simulink model "User_Interface_Unit"  (R2019a)
settings: Solver=ode2  StartTime=0.0  StopTime=inf  FixedStep=0.002  RelTol=1e-3  EnableMultiTasking=on
undefined symbols (not defined in the file): Host
libraries: quarc_library x15, simulink x6
settings Model: Creator=User  LastModifiedBy=mbohra
settings SolverCC: PositivePriorityOrder=on
settings DataIOCC: ReturnWorkspaceOutputs=off
settings DebuggingCC: PregeneratedLibrarySubsystemCodeDiagnostic=none  ArithmeticOperatorsInVariantConditions=warning
settings SFSimCC: SimUseLocalCustomCode=off
settings RTWCC: SystemTargetFile=quarc_linux_nvidia.tlc  TemplateMakefile=quarc_linux_nvidia_tmf  Description=QUARC Linux Nvidia Target  RTWUseLocalCustomCode=off
settings STFCustomTargetCC: TargetLibSuffix=.a  TargetPreCompLibLocation=C:\PROGRA~3\QUARC\lib\2019a\LINUX_~1\release  TargetLangStandard=C99 (ISO)  ConcurrentExecutionCompliant=on  SystemTargetFile=quarc_linux_nvidia.tlc
settings GRTTargetCC: TargetLibSuffix=.a  TargetPreCompLibLocation=C:\PROGRA~3\QUARC\lib\2019a\LINUX_~1\release  ParMdlRefBuildCompliant=off  CompOptLevelCompliant=off  CombineOutputUpdateFcns=off  MatFileLogging=off  CPPClassGenCompliant=off  GRTInterface=on  UseToolchainInfoCompliant=off  ExtMode=on  ExtModeMexFile=quarc_comm  ExtModeMexArgs='-w -d /tmp -uri %u'

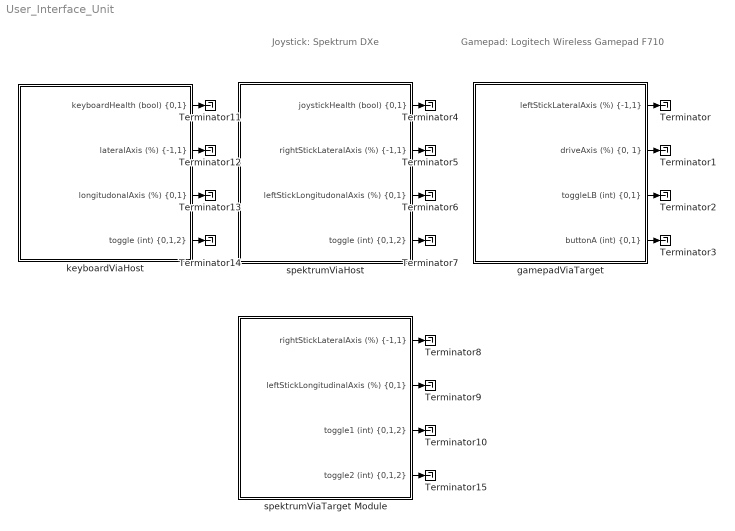
== system User_Interface_Unit ==
  note: Gamepad: Logitech Wireless Gamepad F710
  note: Joystick: Spektrum DXe
  Terminator{,1..15} (16 alike) : Terminator
  gamepadViaTarget : Subsystem
  keyboardViaHost : Subsystem
  spektrumViaHost : Subsystem
  spektrumViaTarget Module : Subsystem
  wires:
  keyboardViaHost/3("longitudonalAxis (%) {0,1}") -> Terminator13/1
  spektrumViaTarget Module/3("toggle1 (int) {0,1,2}") -> Terminator10/1
  spektrumViaHost/2("rightStickLateralAxis (%) {-1,1}") -> Terminator5/1
  spektrumViaTarget Module/2("leftStickLongitudinalAxis (%) {0,1}") -> Terminator9/1
  spektrumViaTarget Module/4("toggle2 (int) {0,1,2}") -> Terminator15/1
  spektrumViaHost/1("joystickHealth (bool) {0,1}") -> Terminator4/1
  spektrumViaTarget Module/1("rightStickLateralAxis (%) {-1,1}") -> Terminator8/1
  spektrumViaHost/3("leftStickLongitudonalAxis (%) {0,1}") -> Terminator6/1
  spektrumViaHost/4("toggle (int) {0,1,2}") -> Terminator7/1
  keyboardViaHost/2("lateralAxis (%) {-1,1}") -> Terminator12/1
  keyboardViaHost/4("toggle (int) {0,1,2}") -> Terminator14/1
  keyboardViaHost/1("keyboardHealth (bool) {0,1}") -> Terminator11/1
  gamepadViaTarget/1("leftStickLateralAxis (%) {-1,1}") -> Terminator/1
  gamepadViaTarget/2("driveAxis (%) {0, 1}") -> Terminator1/1
  gamepadViaTarget/3("toggleLB (int) {0,1}") -> Terminator2/1
  gamepadViaTarget/4("buttonA (int) {0,1}") -> Terminator3/1

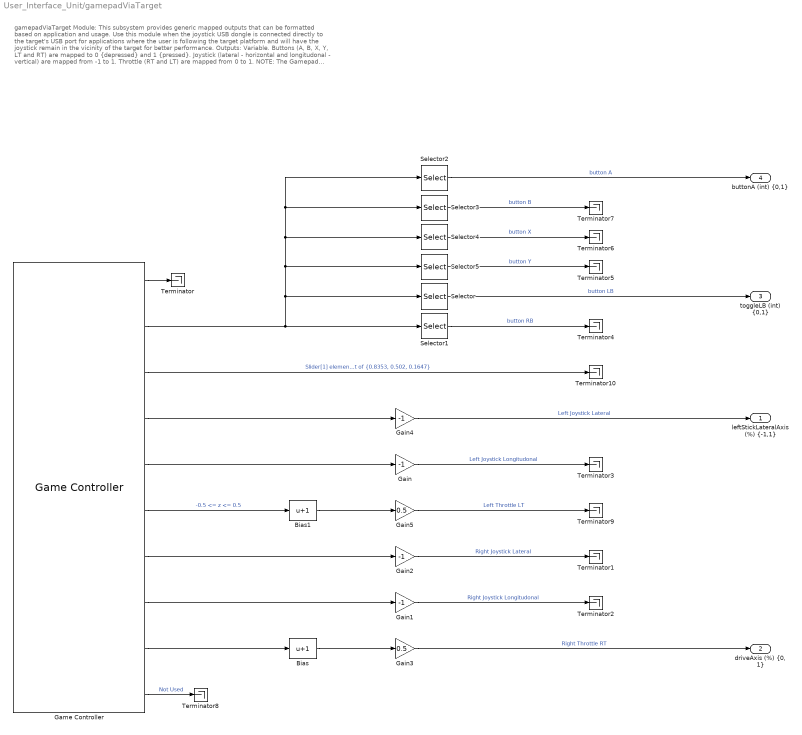
== system User_Interface_Unit/gamepadViaTarget ==
  note: gamepadViaTarget Module:
      |
      | This subsystem provides generic mapped outputs that can be formatted based on application and usage. Use this module when the joystick USB dongle is connected directly to the target's USB port for applications where the user is following the target platform and will have the joystick remain in the vicinity of the target for better performance.
      |
      | Outputs:
      | Variable.
      | Buttons (A, B, X, Y, LT and RT) are mapped to 0 {depressed} and 1 {pressed}.
      | Joystick (lateral - horizontal and longitudonal - vertical) are mapped from -1 to 1.
      | Throttle (RT and LT) are mapped from 0 to 1.
      |
      | NOTE: The Gamepad F710 dongle MUST be plugged into the target's USB port to use this module. Connect the target to a Monitor/Keyboard/Mouse or SSH into the client and run the following command in the terminal:
      | ls -l /dev/input/by-id
      | Find the output with the term ' usb-Logitech_Wireless_Gamepad_F710_XXXXXXX 4-event-joystick ' in it. Find the event number at the end, for example ../event6 , and add 1 to it, for example, 6+1 = 7. Use that as the Controller # in the Game Controller block below.
  Bias : Bias  Bias=1
  Bias1 : Bias  Bias=1
  Gain{,1..2,4} (4 alike) : Gain  Gain=-1
  Gain3 : Gain  Gain=0.5
  Gain5 : Gain  Gain=0.5
  Game Controller : quarc_library/Devices/Peripherals/Target/Game Controller  controller=7  buffer_size=12  deadzone=[]  saturation=[]  sample_time=qc_get_step_size  auto_center=off  enabled=on
      settings: SourceProductName=QUARC Targets
  Selector : Selector  InputPortWidth=32  IndexOptions=Index vector (dialog)  Indices=[5]  OutputSizes=1
  Selector1 : Selector  InputPortWidth=32  IndexOptions=Index vector (dialog)  Indices=[6]  OutputSizes=1
  Selector2 : Selector  InputPortWidth=32  IndexOptions=Index vector (dialog)  Indices=[1]  OutputSizes=1
  Selector3 : Selector  InputPortWidth=32  IndexOptions=Index vector (dialog)  Indices=[2]  OutputSizes=1
  Selector4 : Selector  InputPortWidth=32  IndexOptions=Index vector (dialog)  Indices=[3]  OutputSizes=1
  Selector5 : Selector  InputPortWidth=32  IndexOptions=Index vector (dialog)  Indices=[4]  OutputSizes=1
  Terminator{,1..10} (11 alike) : Terminator
  "leftStickLateralAxis (%) {-1,1}" : Outport
  "driveAxis (%) {0, 1}" : Outport  Port=2
  "toggleLB (int) {0,1}" : Outport  Port=3
  "buttonA (int) {0,1}" : Outport  Port=4
  wires:
  Selector1/1 -> Terminator4/1  "button RB"
  Gain/1 -> Terminator3/1  "Left Joystick Longitudonal"
  Gain1/1 -> Terminator2/1  "Right Joystick Longitudonal"
  Gain2/1 -> Terminator1/1  "Right Joystick Lateral"
  Selector2/1 -> "buttonA (int) {0,1}"/1  "button A"
  Gain4/1 -> "leftStickLateralAxis (%) {-1,1}"/1  "Left Joystick Lateral"
  Gain3/1 -> "driveAxis (%) {0, 1}"/1  "Right Throttle RT"
  Bias/1 -> Gain3/1
  Game Controller/9 -> Bias/1
  Selector/1 -> "toggleLB (int) {0,1}"/1  "button LB"
  Game Controller/2 -> Selector4/1, Selector3/1, Selector2/1, Selector5/1, Selector/1, Selector1/1
  Game Controller/7 -> Gain2/1
  Game Controller/8 -> Gain1/1
  Game Controller/4 -> Gain4/1
  Game Controller/5 -> Gain/1
  Game Controller/1 -> Terminator/1
  Selector3/1 -> Terminator7/1  "button B"
  Selector4/1 -> Terminator6/1  "button X"
  Selector5/1 -> Terminator5/1  "button Y"
  Game Controller/10 -> Terminator8/1  "Not Used"
  Game Controller/6 -> Bias1/1  "-0.5 <= z <= 0.5"
  Bias1/1 -> Gain5/1
  Gain5/1 -> Terminator9/1  "Left Throttle LT"
  Game Controller/3 -> Terminator10/1  "Slider[1] element of {0.8353, 0.502, 0.1647}"

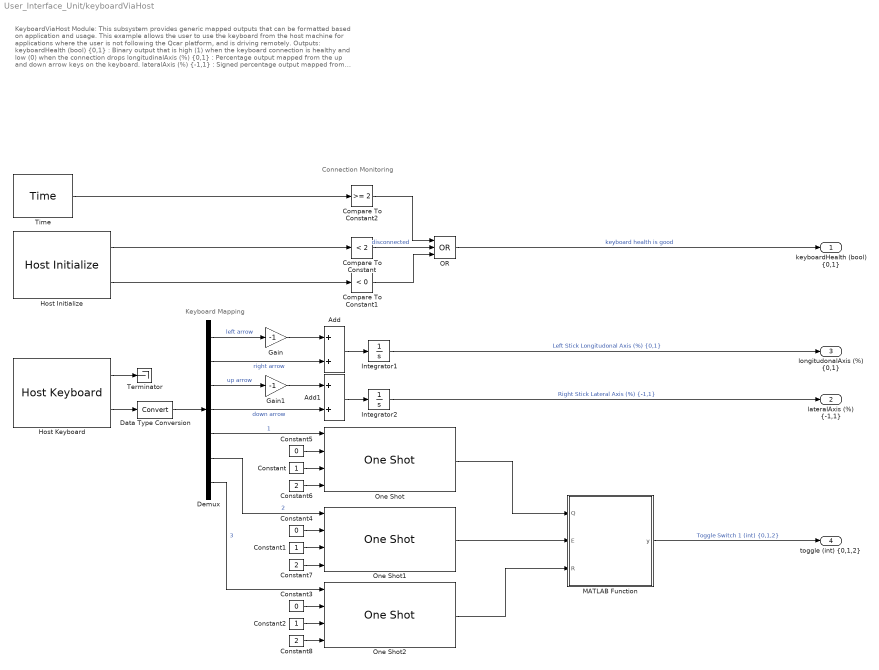
== system User_Interface_Unit/keyboardViaHost ==
  note: Connection Monitoring
  note: KeyboardViaHost Module:
      |
      | This subsystem provides generic mapped outputs that can be formatted based on application and usage. This example allows the user to use the keyboard from the host machine for applications where the user is not following the Qcar platform, and is driving remotely.
      |
      | Outputs:
      | keyboardHealth (bool) {0,1} : Binary output that is high (1) when the keyboard connection is healthy and low (0) when the connection drops
      | longitudinalAxis (%) {0,1} : Percentage output mapped from the up and down arrow keys on the keyboard.
      | lateralAxis (%) {-1,1} : Signed percentage output mapped from the left and right arrow keys on the keyboard.
      | toggle (int) {0,1,2} : 3-state output mapped from the 1, 2, 3 alpha-numeric keys (NOT on the NUMPAD).
      |
      | Note: Holding the arrow keys longer will increase/decrease the value further. Releasing the key will maintain values.
  note: Keyboard Mapping
  Add : Sum
  Add1 : Sum
  Compare To Constant : simulink/Logic and Bit Operations/Compare To Constant  relop=<  const=2  OutDataTypeStr=boolean
  Compare To Constant1 : simulink/Logic and Bit Operations/Compare To Constant  relop=<  const=0  OutDataTypeStr=boolean
  Compare To Constant2 : simulink/Logic and Bit Operations/Compare To Constant  relop=>=  const=2  OutDataTypeStr=boolean
  Constant : Constant
  Constant1 : Constant
  Constant2 : Constant
  Constant3 : Constant  Value=0
  Constant4 : Constant  Value=0
  Constant5 : Constant  Value=0
  Constant6 : Constant  Value=2
  Constant7 : Constant  Value=2
  Constant8 : Constant  Value=2
  Data Type Conversion : DataTypeConversion
  Demux : Demux  Outputs=7
  Gain : Gain  Gain=-1
  Gain1 : Gain  Gain=-1
  Host Initialize : quarc_library/Devices/Peripherals/Host/Host Initialize  object_name=Host-2  uri_source=Use external mode communications  uri=tcpip://localhost:18001  apply_uri_to_all_configs=on  send_buffer_size=1000  receive_buffer_size=1000  thread_priority=0  run_client=on  use_window=off  window_position=[]  sample_time=qc_get_step_size  active=on
      settings: SourceProductName=QUARC Targets
  Host Keyboard : quarc_library/Devices/Peripherals/Host/Host Keyboard  object_name=Host-2  virtual_key="[37  39  40  38  49  50  51]"  sample_time=qc_get_step_size  enabled=on  debug_mode=off
      settings: SourceProductName=QUARC Targets
  Integrator1 : Integrator  LimitOutput=on  UpperSaturationLimit=1  LowerSaturationLimit=0
  Integrator2 : Integrator  LimitOutput=on  UpperSaturationLimit=1  LowerSaturationLimit=-1
  MATLAB Function : MATLAB Function  TreatAsAtomicUnit=on
  OR : Logic  Operator=OR  Inputs=3  IconShape=distinctive  AllPortsSameDT=off  OutDataTypeStr=boolean
  One Shot : quarc_library/Discontinuities/One Shot  trigger_type=Rising edge  redun_pulse=Ignore extraneous pulse  width_source=External input port  pulse_width=100
      settings: SourceProductName=QUARC Targets
  One Shot1 : quarc_library/Discontinuities/One Shot  trigger_type=Rising edge  redun_pulse=Ignore extraneous pulse  width_source=External input port  pulse_width=100
      settings: SourceProductName=QUARC Targets
  One Shot2 : quarc_library/Discontinuities/One Shot  trigger_type=Rising edge  redun_pulse=Ignore extraneous pulse  width_source=External input port  pulse_width=100
      settings: SourceProductName=QUARC Targets
  Terminator : Terminator
  Time : quarc_library/Sources/Time/Time  time_source=Wall clock  sample_time=qc_get_step_size
  "keyboardHealth (bool) {0,1}" : Outport
  "lateralAxis (%) {-1,1}" : Outport  Port=2
  "longitudonalAxis (%) {0,1}" : Outport  Port=3
  "toggle (int) {0,1,2}" : Outport  Port=4
  wires:
  Integrator1/1 -> "longitudonalAxis (%) {0,1}"/1  "Left Stick Longitudonal Axis (%) {0,1}"
  One Shot/1 -> MATLAB Function/1(Q)
  Constant2/1 -> One Shot2/3
  Host Initialize/1 -> Compare To Constant/1
  Constant/1 -> One Shot/3
  Constant6/1 -> One Shot/4
  Demux/2 -> Add/2  "right arrow"
  One Shot1/1 -> MATLAB Function/2(E)
  Compare To Constant/1 -> OR/2  "disconnected"
  One Shot2/1 -> MATLAB Function/3(R)
  Integrator2/1 -> "lateralAxis (%) {-1,1}"/1  "Right Stick Lateral Axis (%) {-1,1}"
  Demux/1 -> Gain/1  "left arrow"
  Constant3/1 -> One Shot2/2
  Constant8/1 -> One Shot2/4
  Host Keyboard/2 -> Data Type Conversion/1
  Gain1/1 -> Add1/1
  OR/1 -> "keyboardHealth (bool) {0,1}"/1  "keyboard health is good"
  Demux/7 -> One Shot2/1  "3"
  Constant4/1 -> One Shot1/2
  Constant1/1 -> One Shot1/3
  Demux/5 -> One Shot/1  "1"
  Compare To Constant2/1 -> OR/1
  Time/1 -> Compare To Constant2/1
  Host Keyboard/1 -> Terminator/1
  Add1/1 -> Integrator2/1
  Gain/1 -> Add/1
  Constant5/1 -> One Shot/2
  Add/1 -> Integrator1/1
  Constant7/1 -> One Shot1/4
  Compare To Constant1/1 -> OR/3
  Data Type Conversion/1 -> Demux/1
  Host Initialize/2 -> Compare To Constant1/1
  MATLAB Function/1(y) -> "toggle (int) {0,1,2}"/1  "Toggle Switch 1 (int) {0,1,2}"
  Demux/3 -> Gain1/1  "up arrow"
  Demux/4 -> Add1/2  "down arrow"
  Demux/6 -> One Shot1/1  "2"

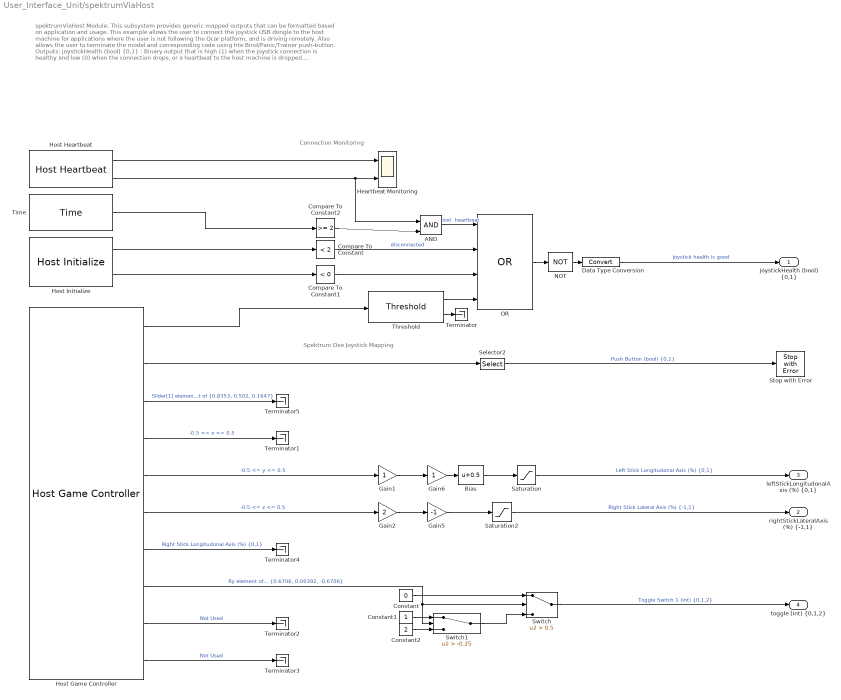
== system User_Interface_Unit/spektrumViaHost ==
  note: Connection Monitoring
  note: Spektrum Dxe Joystick Mapping
  note: spektrumViaHost Module:
      |
      | This subsystem provides generic mapped outputs that can be formatted based on application and usage. This example allows the user to connect the joystick USB dongle to the host machine for applications where the user is not following the Qcar platform, and is driving remotely. Also allows the user to terminate the model and corresponding code using hte Bind/Panic/Trainer push-button.
      |
      | Outputs:
      | joystickHealth (bool) {0,1} : Binary output that is high (1) when the joystick connection is healthy and low (0) when the connection drops, or a heartbeat to the host machine is dropped.
      | leftStickLongitudinalAxis (%) {0,1} : Percentage output mapped from the left stick of the joystick in the longitudinal axis
      | rightStickLateralAxis (%) {-1,1} : Signed percentage output mapped from the right stick of the joystick in the lateral axis
      | toggle (int) {0,1,2} : 3-state output mapped from the joystick's first toggle (labelled Flight Mode)
      |
      | NOTE: The Spektrum Joystick USB Dongle MUST be plugged into the Host PC's USB port to use this module. Open the Host Game Controller block below, and in the Controller number menu, select the one with the SPEKTRUM RECEIVER label next to it.
  AND : Logic  IconShape=distinctive  AllPortsSameDT=off  OutDataTypeStr=boolean
  Bias : Bias  Bias=0.5
  Compare To Constant : simulink/Logic and Bit Operations/Compare To Constant  relop=<  const=2  OutDataTypeStr=boolean
  Compare To Constant1 : simulink/Logic and Bit Operations/Compare To Constant  relop=<  const=0  OutDataTypeStr=boolean
  Compare To Constant2 : simulink/Logic and Bit Operations/Compare To Constant  relop=>=  const=2  OutDataTypeStr=boolean
  Constant : Constant  Value=0
  Constant1 : Constant
  Constant2 : Constant  Value=2
  Data Type Conversion : DataTypeConversion
  Gain1 : Gain
  Gain2 : Gain  Gain=2
  Gain5 : Gain  Gain=-1
  Gain6 : Gain
  Heartbeat Monitoring : Scope  NumInputPorts=2
  Host Game Controller : quarc_library/Devices/Peripherals/Host/Host Game Controller  object_name=Host-1  controller=1  buffer_size=12  deadzone=[]  saturation=[]  sample_time=qc_get_step_size  auto_center=off  enabled=off  debug_mode=off
      settings: SourceProductName=QUARC Targets
  Host Heartbeat : quarc_library/Devices/Peripherals/Host/Host Heartbeat  object_name=Host-1  period=0.1  loss_interval=0.5  sample_time=qc_get_step_size  enabled=off
      settings: SourceProductName=QUARC Targets
  Host Initialize : quarc_library/Devices/Peripherals/Host/Host Initialize  object_name=Host-1  uri_source=Specify via dialog (do not evaluate)  uri=tcpip://%h:18001  apply_uri_to_all_configs=on  send_buffer_size=1000  receive_buffer_size=1000  thread_priority=0  run_client=on  use_window=off  window_position=[]  sample_time=qc_get_step_size  active=on
      settings: AttributesFormatString="\"tcpip://linuxdev:18001\""  SourceProductName=QUARC Targets
  NOT : Logic  Operator=NOT  IconShape=distinctive  AllPortsSameDT=off  OutDataTypeStr=boolean
  OR : Logic  Operator=OR  Inputs=4  IconShape=distinctive  AllPortsSameDT=off  OutDataTypeStr=boolean
  Saturation : Saturate  UpperLimit=1  LowerLimit=0
  Saturation2 : Saturate  UpperLimit=1  LowerLimit=-1
  Selector2 : Selector  InputPortWidth=32  IndexOptions=Index vector (dialog)  Indices=[1]  OutputSizes=1
  Stop with Error : quarc_library/Sinks/Error Handling/Stop with Error  message_type=Fixed error message  message=Emergency Stop Issued
      settings: AttributesFormatString="\"%<message>\""  SourceProductName=QUARC Targets
  Switch : Switch  Criteria=u2 > Threshold  Threshold=0.5
  Switch1 : Switch  Criteria=u2 > Threshold  Threshold=-0.25
  Terminator{,1..5} (6 alike) : Terminator
  Threshold : quarc_library/Discontinuities/Threshold  operator=<=  param_src=Specify via dialog  threshold=0  duration=2
      settings: SourceProductName=QUARC Targets
  Time : quarc_library/Sources/Time/Time  time_source=Wall clock  sample_time=qc_get_step_size
  "joystickHealth (bool) {0,1}" : Outport
  "rightStickLateralAxis (%) {-1,1}" : Outport  Port=2
  "leftStickLongitudonalAxis (%) {0,1}" : Outport  Port=3
  "toggle (int) {0,1,2}" : Outport  Port=4
  wires:
  Constant/1 -> Switch/1
  Host Game Controller/9 -> Terminator2/1  "Not Used"
  Host Game Controller/2 -> Selector2/1
  Host Game Controller/8 -> Switch1/2, Switch/2  "Ry element of {0.6706, 0.00392, -0.6706}"
  Constant1/1 -> Switch1/1
  Switch1/1 -> Switch/3
  Host Game Controller/5 -> Gain1/1  "-0.5 <= y <= 0.5"
  Saturation/1 -> "leftStickLongitudonalAxis (%) {0,1}"/1  "Left Stick Longitudonal Axis (%) {0,1}"
  Compare To Constant2/1 -> AND/2
  Switch/1 -> "toggle (int) {0,1,2}"/1  "Toggle Switch 1 (int) {0,1,2}"
  Bias/1 -> Saturation/1
  Gain5/1 -> Saturation2/1
  Host Heartbeat/2 -> AND/1, Heartbeat Monitoring/2
  Gain1/1 -> Gain6/1
  Saturation2/1 -> "rightStickLateralAxis (%) {-1,1}"/1  "Right Stick Lateral Axis (%) {-1,1}"
  Time/1 -> Compare To Constant2/1
  Host Game Controller/4 -> Terminator1/1  "-0.5 <= x <= 0.5"
  Compare To Constant/1 -> OR/2  "disconnected"
  Host Game Controller/3 -> Terminator5/1  "Slider[1] element of {0.8353, 0.502, 0.1647}"
  Host Game Controller/6 -> Gain2/1  "-0.5 <= z <= 0.5"
  Gain2/1 -> Gain5/1
  Data Type Conversion/1 -> "joystickHealth (bool) {0,1}"/1  "joystick health is good"
  OR/1 -> NOT/1
  Gain6/1 -> Bias/1
  Threshold/1 -> OR/4
  Host Heartbeat/1 -> Heartbeat Monitoring/1
  Host Game Controller/7 -> Terminator4/1  "Right Stick Longitudonal Axis (%) {0,1}"
  AND/1 -> OR/1  "lost  heartbeat"
  Threshold/2 -> Terminator/1
  Host Game Controller/1 -> Threshold/1
  Compare To Constant1/1 -> OR/3
  Host Game Controller/10 -> Terminator3/1  "Not Used"
  Constant2/1 -> Switch1/3
  Host Initialize/2 -> Compare To Constant1/1
  Host Initialize/1 -> Compare To Constant/1
  Selector2/1 -> Stop with Error/1  "Push Button (bool) {0,1}"
  NOT/1 -> Data Type Conversion/1

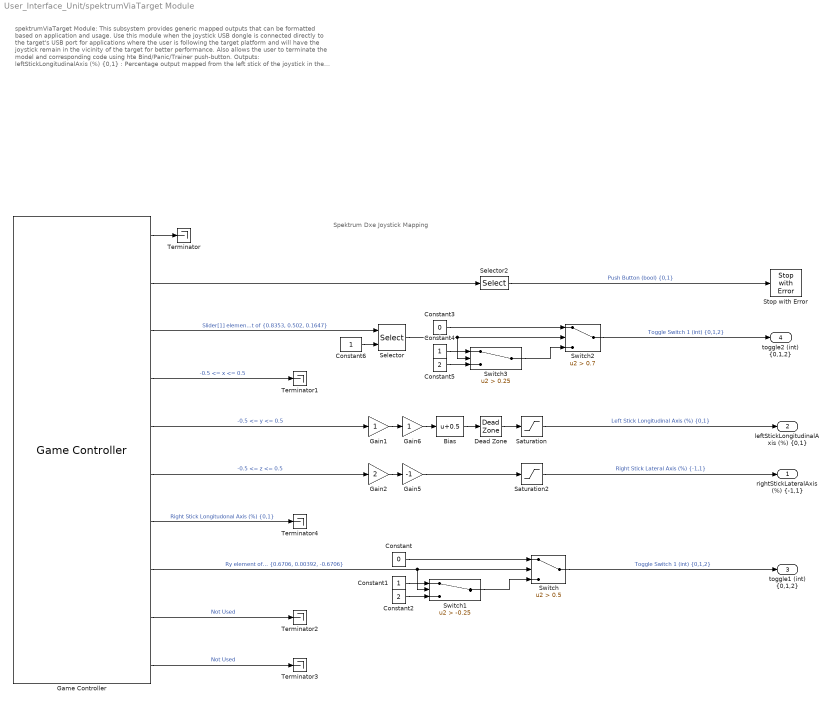
== system User_Interface_Unit/spektrumViaTarget Module ==
  note: spektrumViaTarget Module:
      |
      | This subsystem provides generic mapped outputs that can be formatted based on application and usage. Use this module when the joystick USB dongle is connected directly to the target's USB port for applications where the user is following the target platform and will have the joystick remain in the vicinity of the target for better performance. Also allows the user to terminate the model and corresponding code using hte Bind/Panic/Trainer push-button.
      |
      | Outputs:
      | leftStickLongitudinalAxis (%) {0,1} : Percentage output mapped from the left stick of the joystick in the longitudinal axis
      | rightStickLateralAxis (%) {-1,1} : Signed percentage output mapped from the right stick of the joystick in the lateral axis
      | toggle1 (int) {0,1,2} : 3-state output mapped from the joystick's first toggle
      | toggle2 (int) {0,1,2} : 3-state output mapped from the joystick's second toggle
      |
      | NOTE: The Spektrum Joystick USB Dongle MUST be plugged into the QCar's USB port to use this module. Connect the QCar to a Monitor/Keyboard/Mouse or SSH into the client and run the following command in the terminal:
      | ls -l /dev/input/by-id
      | Find the output with the term ' usb-Horizon_Hobby_SPEKTRUM_RECEIVER_00000000001A-event-joystick ' in it. Find the event number at the end, for example ../event4 , and add 1 to it, for example, 4+1 = 5. Use that as the Controller # in the Game Controller block below.
  note: Spektrum Dxe Joystick Mapping
  Bias : Bias  Bias=0.5
  Constant : Constant  Value=0
  Constant1 : Constant
  Constant2 : Constant  Value=2
  Constant3 : Constant  Value=0
  Constant4 : Constant
  Constant5 : Constant  Value=2
  Constant6 : Constant
  Dead Zone : DeadZone  LowerValue=-0.1  UpperValue=0.1  SaturateOnIntegerOverflow=on
  Gain1 : Gain
  Gain2 : Gain  Gain=2
  Gain5 : Gain  Gain=-1
  Gain6 : Gain
  Game Controller : quarc_library/Devices/Peripherals/Target/Game Controller  controller=1  buffer_size=12  deadzone=[]  saturation=[]  sample_time=qc_get_step_size  auto_center=off  enabled=on
      settings: SourceProductName=QUARC Targets
  Saturation : Saturate  UpperLimit=1  LowerLimit=0
  Saturation2 : Saturate  UpperLimit=1  LowerLimit=-1
  Selector : Selector  InputPortWidth=2  IndexOptions=Index vector (port)  Indices=[1 3]  OutputSizes=1
  Selector2 : Selector  InputPortWidth=32  IndexOptions=Index vector (dialog)  Indices=[1]  OutputSizes=1
  Stop with Error : quarc_library/Sinks/Error Handling/Stop with Error  message_type=Fixed error message  message=Emergency Stop Issued
      settings: AttributesFormatString="\"%<message>\""  SourceProductName=QUARC Targets
  Switch : Switch  Criteria=u2 > Threshold  Threshold=0.5
  Switch1 : Switch  Criteria=u2 > Threshold  Threshold=-0.25
  Switch2 : Switch  Criteria=u2 > Threshold  Threshold=0.7
  Switch3 : Switch  Criteria=u2 > Threshold  Threshold=0.25
  Terminator{,1..4} (5 alike) : Terminator
  "rightStickLateralAxis (%) {-1,1}" : Outport
  "leftStickLongitudinalAxis (%) {0,1}" : Outport  Port=2
  "toggle1 (int) {0,1,2}" : Outport  Port=3
  "toggle2 (int) {0,1,2}" : Outport  Port=4
  wires:
  Selector/1 -> Switch3/2, Switch2/2
  Switch3/1 -> Switch2/3
  Constant4/1 -> Switch3/1
  Bias/1 -> Dead Zone/1
  Switch/1 -> "toggle1 (int) {0,1,2}"/1  "Toggle Switch 1 (int) {0,1,2}"
  Switch2/1 -> "toggle2 (int) {0,1,2}"/1  "Toggle Switch 1 (int) {0,1,2}"
  Game Controller/1 -> Terminator/1
  Constant3/1 -> Switch2/1
  Game Controller/6 -> Gain2/1  "-0.5 <= z <= 0.5"
  Constant5/1 -> Switch3/3
  Constant6/1 -> Selector/2
  Constant/1 -> Switch/1
  Switch1/1 -> Switch/3
  Game Controller/7 -> Terminator4/1  "Right Stick Longitudonal Axis (%) {0,1}"
  Game Controller/8 -> Switch1/2, Switch/2  "Ry element of {0.6706, 0.00392, -0.6706}"
  Dead Zone/1 -> Saturation/1
  Game Controller/10 -> Terminator3/1  "Not Used"
  Gain6/1 -> Bias/1
  Gain2/1 -> Gain5/1
  Saturation2/1 -> "rightStickLateralAxis (%) {-1,1}"/1  "Right Stick Lateral Axis (%) {-1,1}"
  Selector2/1 -> Stop with Error/1  "Push Button (bool) {0,1}"
  Game Controller/5 -> Gain1/1  "-0.5 <= y <= 0.5"
  Game Controller/4 -> Terminator1/1  "-0.5 <= x <= 0.5"
  Game Controller/3 -> Selector/1  "Slider[1] element of {0.8353, 0.502, 0.1647}"
  Gain5/1 -> Saturation2/1
  Saturation/1 -> "leftStickLongitudinalAxis (%) {0,1}"/1  "Left Stick Longitudinal Axis (%) {0,1}"
  Constant1/1 -> Switch1/1
  Game Controller/2 -> Selector2/1
  Gain1/1 -> Gain6/1
  Game Controller/9 -> Terminator2/1  "Not Used"
  Constant2/1 -> Switch1/3

== matlab function User_Interface_Unit/keyboardViaHost/MATLAB Function ==
  data: Q input; E input; y output; R input
function y = fcn(Q, E, R)

persistent prev
if isempty(prev)
    prev = 1;
end
y = prev;

if E > 0
    y = 1;
elseif Q > 0
    y = 0;
elseif R > 0
    y = 2;
end

prev = y;
